simulink model "Anstellwinkelschwingung"  (R2021b)
settings: Solver=ode4  StartTime=0.0  StopTime=15.0  FixedStep=0.02  RelTol=1e-3
undefined symbols (not defined in the file): BFZ, NickD
settings Model: Creator=jonih  LastModifiedBy=jonih

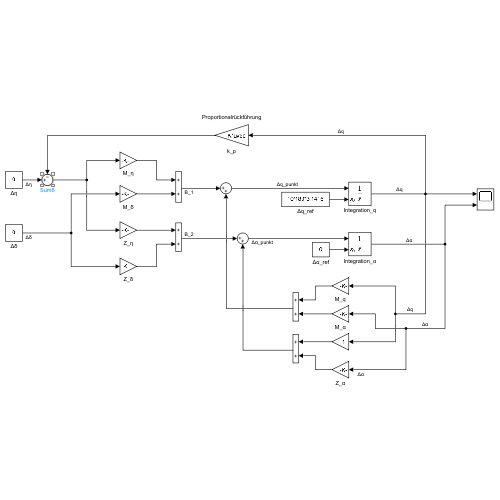
[thumbnail: Simulink's stored preview of the top-level diagram]
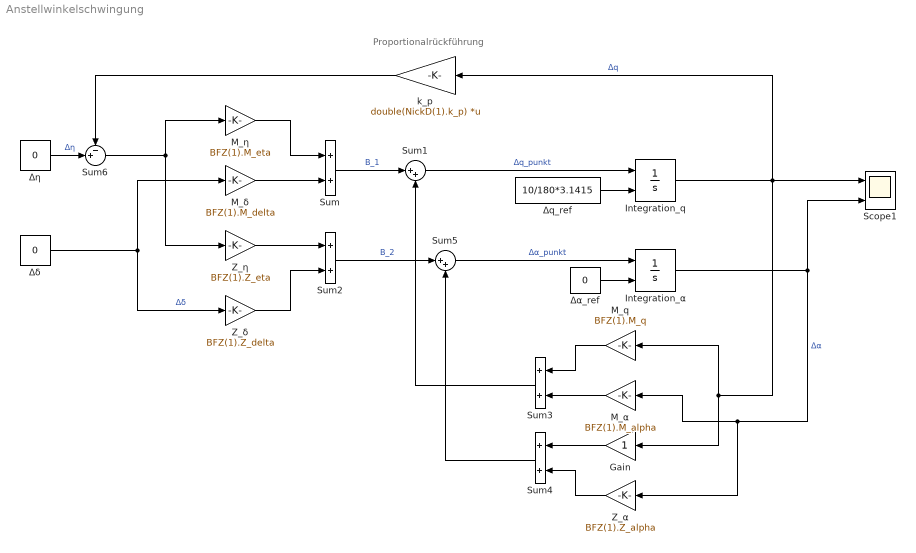
== system Anstellwinkelschwingung ==
  note: Proportionalrückführung
  Gain : Gain
  Integration_q : Integrator  InitialConditionSource=external
  Integration_α : Integrator  InitialConditionSource=external
  M_q : Gain  Gain=BFZ(1).M_q
  M_α : Gain  Gain=BFZ(1).M_alpha
  M_δ : Gain  Gain=BFZ(1).M_delta
  M_η : Gain  Gain=BFZ(1).M_eta
  Scope1 : Scope  NumInputPorts=2
  Sum{,2..4} (4 alike) : Sum
  Sum1 : Sum  Inputs=|++
  Sum5 : Sum  Inputs=|++
  Sum6 : Sum  Inputs=-+|
  Z_α : Gain  Gain=BFZ(1).Z_alpha
  Z_δ : Gain  Gain=BFZ(1).Z_delta
  Z_η : Gain  Gain=BFZ(1).Z_eta
  k_p : Gain  Gain=double(NickD(1).k_p)  Multiplication=Matrix(K*u) (u vector)
  Δq_ref : Constant  Value=10/180*3.1415
  Δα_ref : Constant  Value=0
  Δδ : Constant  Value=0
  Δη : Constant  Value=0
  wires:
  Sum1/1 -> Integration_q/1  "Δq_punkt"
  Integration_q/1 -> k_p/1, Gain/1, M_q/1, Scope1/1  "Δq"
  Δη/1 -> Sum6/2  "Δη"
  Δδ/1 -> Z_δ/1, M_δ/1  "Δδ"
  Sum/1 -> Sum1/1  "B_1"
  Sum2/1 -> Sum5/1  "B_2"
  Sum3/1 -> Sum1/2
  Sum4/1 -> Sum5/2
  Δq_ref/1 -> Integration_q/2
  Z_δ/1 -> Sum2/2
  M_δ/1 -> Sum/2
  Z_η/1 -> Sum2/1
  M_η/1 -> Sum/1
  Gain/1 -> Sum4/1
  Z_α/1 -> Sum4/2
  M_q/1 -> Sum3/1
  M_α/1 -> Sum3/2
  Δα_ref/1 -> Integration_α/2
  Sum5/1 -> Integration_α/1  "Δα_punkt"
  Integration_α/1 -> Scope1/2, Z_α/1, M_α/1  "Δα"
  k_p/1 -> Sum6/1
  Sum6/1 -> Z_η/1, M_η/1
